simulink model "wind_prili"  (R2021a)
settings: Solver=VariableStepAuto  StartTime=0.0  StopTime=10.0  RelTol=1e-3
undefined symbols (not defined in the file): D1, Delta
libraries: spsThreePhaseVIMeasurementLib x3, spsThreePhaseParallelRLCLoadLib x2, spsPower3phInstantaneousLib x2, spsThreePhaseSourceLib x1, spsExcitationSystemLib x1, spsSynchronousMachinepuStandardLib x1, spsThreePhaseTransformerTwoWindingsLib x1, spsWindTurbineLib x1, spspowerguiLib x1
settings Model: Creator=HP  LastModifiedBy=HP

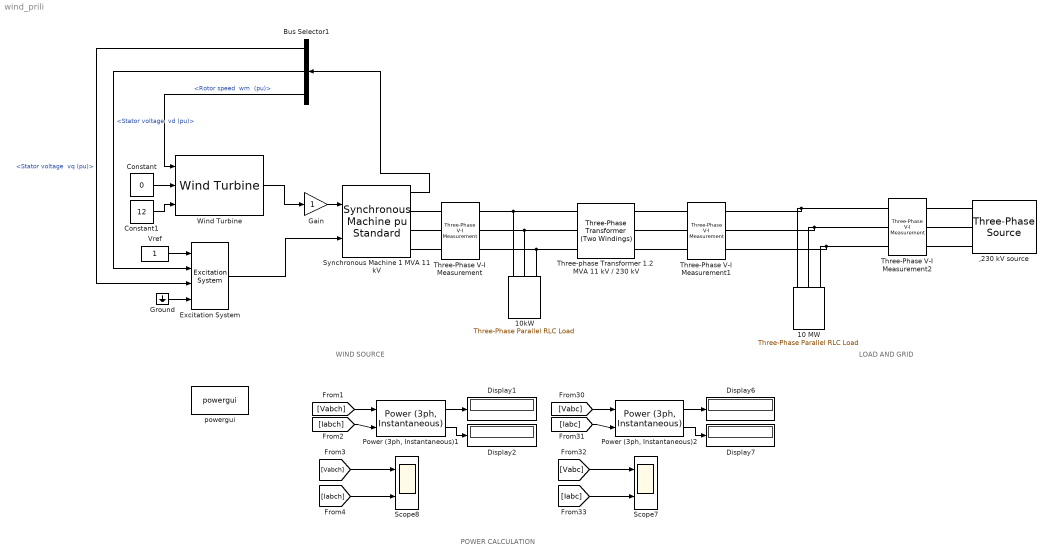
== system wind_prili ==
  note: LOAD AND GRID
  note: WIND SOURCE
  note: POWER CALCULATION
  ,230 kV source : spsThreePhaseSourceLib/Three-Phase Source  InternalConnection=Yg  VoltagePhases=off  Voltage=230e3  PhaseAngle=0  Voltage_phases=[25e3 25e3 25e3]/sqrt(3)  PhaseAngles_phases=[0 -120 +120]  Frequency=50  NonIdealSource=on  SpecifyImpedance=off  Resistance=0.529  Inductance=0.0140  ShortCircuitLevel=10000e6  BaseVoltage=230e3  XRratio=10  BusType=swing  Pref=0  Qref=0  Prefabc=[10e3, 10e3, 10e3]  Qrefabc=[0, 0, 0]  Qmin=-Inf  Qmax=Inf
  10 MW : spsThreePhaseParallelRLCLoadLib/Three-Phase Parallel RLC Load  LConnTagsString=A|B|C  Configuration=Y (grounded)  NominalVoltage=230e3  Vabc=[1e3 1e3 1e3]  Vabcp=[1e3 1e3 1e3]  NominalFrequency=50  UnbalancedPower=off  ActivePower=1.8e6  InductivePower=0.8e6  CapacitivePower=0  Pabc=[10e3 9e3 11e3]  QLabc=[100 90 110]  QCabc=[100 90 110]  Pabcp=[10e3 9e3 11e3]  QLabcp=[100 90 110]  QCabcp=[100 90 110]  Measurements=None  LoadType=constant Z
  10kW : spsThreePhaseParallelRLCLoadLib/Three-Phase Parallel RLC Load  LConnTagsString=A|B|C  Configuration=Y (grounded)  NominalVoltage=11e3  Vabc=[1e3 1e3 1e3]  Vabcp=[1e3 1e3 1e3]  NominalFrequency=50  UnbalancedPower=off  ActivePower=10e3  InductivePower=0  CapacitivePower=0  Pabc=[10e3 9e3 11e3]  QLabc=[100 90 110]  QCabc=[100 90 110]  Pabcp=[10e3 9e3 11e3]  QLabcp=[100 90 110]  QCabcp=[100 90 110]  Measurements=None  LoadType=constant Z
  Bus Selector1 : BusSelector  OutputSignals="dq0 components.Stator voltage  vq (pu),dq0 components.Stator voltage  vd (pu),Mechanical.Rotor speed  wm  (pu)"
  Constant : Constant  Value=0
  Constant1 : Constant  Value=12
  Display{1..2,6..7} (4 alike) : Display
  Excitation System : spsExcitationSystemLib/Excitation System  tr=20e-3  reg=[ 300, 0.001 ]  exc=[ 1, 0 ]  tgr=[ 0, 0 ]  damp=[ 0.001, 0.1 ]  sat=[ 0, 0 ]  lim=[ -11.5, 11.5, 0 ]  v0=[1,1.26864]
      settings: SourceProductBaseCode=PS
  Gain : Gain
  Ground : Ground
  "Power (3ph, Instantaneous)1" : spsPower3phInstantaneousLib/Power (3ph, Instantaneous)
  "Power (3ph, Instantaneous)2" : spsPower3phInstantaneousLib/Power (3ph, Instantaneous)
  Scope7 : Scope  NumInputPorts=2
  Scope8 : Scope  NumInputPorts=2
  Synchronous Machine 1 MVA 11 kV : spsSynchronousMachinepuStandardLib/Synchronous Machine pu Standard  PresetModel=No  MechanicalLoad=Mechanical power Pm  ShowDetailedParameters=on  RotorType=Salient-pole  Units=per unit standard parameters  MeasurementBus=off  NominalParameters="[ 1E6  11e3   50 ]"  Reactances1=[ 31 32 33 34 35 36 37 ]  Reactances2=[ 1.305, 0.296, 0.252, 0.474, 0.243, 0.18 ]  dAxisTimeConstants=Short-circuit  qAxisTimeConstants=Open-circuit  TimeConstants1=[]  TimeConstants2=[]  TimeConstants3=[]  TimeConstants4=[]  TimeConstants5=[ 1.01, 0.053, 0.1 ]  TimeConstants6=[]  TimeConstants7=[]  TimeConstants8=[]  StatorResistance=2.8544e-3  Mechanical=[ 3.2 0 2]  PolePairs=2  InitialConditions=[0 -83.6958 0.750005 0.750005 0.750005 -13.0459 -133.046 106.954 1.26864]  SetSaturation=off  Saturation=[0.6404,0.7127,0.8441,0.9214,0.9956,1.082,1.19,1.316,1.457;0.7,0.7698,0.8872,0.9466,0.9969,1.046,1.1,1.151,1.201]  LoadFlowParameters=[1 150000000 0 0]  TsPowergui=0  TsBlock=-1  IterativeModel=Trapezoidal non iterative  IterativeDiscreteModel=Trapezoidal non iterative  BusType=PV  Pref=150000000  Qref=0  Qmin=-Inf  Qmax=Inf  PLF=0  QLF=0
      settings: SourceProductBaseCode=PS
  Three-Phase V-I Measurement : spsThreePhaseVIMeasurementLib/Three-Phase V-I Measurement  VoltageMeasurement=phase-to-ground  SetLabelV=on  LabelV=Vabc_w  Vpu=off  VpuLL=off  CurrentMeasurement=no  SetLabelI=off  LabelI=Iabc  Ipu=off  Pbase=100e6  Vbase=500e3  OutputType=Complex  PhasorSimulation=off  PSBequivalent=0
  Three-Phase V-I Measurement1 : spsThreePhaseVIMeasurementLib/Three-Phase V-I Measurement  VoltageMeasurement=phase-to-ground  SetLabelV=on  LabelV=Vabch  Vpu=off  VpuLL=off  CurrentMeasurement=yes  SetLabelI=on  LabelI=Iabch  Ipu=off  Pbase=100e6  Vbase=500e3  OutputType=Complex  PhasorSimulation=off  PSBequivalent=0
  Three-Phase V-I Measurement2 : spsThreePhaseVIMeasurementLib/Three-Phase V-I Measurement  VoltageMeasurement=phase-to-ground  SetLabelV=on  LabelV=Vabc  Vpu=off  VpuLL=off  CurrentMeasurement=yes  SetLabelI=on  LabelI=Iabc  Ipu=off  Pbase=100e6  Vbase=500e3  OutputType=Complex  PhasorSimulation=off  PSBequivalent=0
  Three-phase Transformer 1.2 MVA 11 kV / 230 kV : spsThreePhaseTransformerTwoWindingsLib/Three-Phase Transformer (Two Windings)  Winding1Connection=Delta (D1)  Winding2Connection=Yg  CoreType=Three single-phase transformers  SetSaturation=off  Hysteresis=off  DataFile='hysteresis'  SetInitialFlux=off  Measurements=None  UNITS=pu  NominalPower=[ 1.2e6 50 ]  Winding1="[ 11e3 0.0027  0.08]"  Winding2=[ 230e3 0.0027 0.08]  Rm=500  Lm=500  L0=0.5  Saturation="[ 0,0  ;  0.005,1.2  ;  1.0,1.4 ]"  InitialFluxes=[ 0.8 , -0.8 , 0.7 ]  BreakLoop=off  DiscreteSolver=Trapezoidal iterative  DataType=off  TransfoNumber=0
  Vref : Constant
  Wind Turbine : spsWindTurbineLib/Wind Turbine  Pnom=10e6  Pelec_base=10e6/0.9  wind_base=12  P_wind_base=0.8  speed_nom=1.2  pitch_angle=0  c1_c6="[0.51763          116          0.4            5           21     0.006795]"  cp_nom=0.48  lambda_nom=8.1
      link override Gain: Gain=1
      settings: SourceProductBaseCode=PS
  powergui : spspowerguiLib/powergui  Priority=2  SimulationMode=Continuous  SampleTime=0  frequency=60  Iterations=50  frequencyindice=50  Pbase=100e6  ErrMax=0.0001  UnitsV=kV  UnitsW=MW  buscounter=0  FunctionMessages=off  echomessages=off  EnableUseOfTLC=off  CurrentSourceSwitches=off  DisableSnubberDevices=off  DisableRonSwitches=off  DisableVfSwitches=off  DisplayEquations=off  AutomaticDiscreteSolvers=off  SolverType=Tustin  Interpol=off  ExternalGateDelay=off  methode=off  Ts=0  x0status=blocks  SPID=on  SwTol=0  HookPort=off  NonlinearTolerance=1e-4  nMaxIteration=100  ContinueOnMaxIteration=off  RestoreLinks=warning  ResistiveCurrentMeasurement=off  Frange=logspace(0,3,50)  Ylog=off  Xlog=off  ShowGrid=off  save=off  variable=ZData  structure=0  ZoomFFT=on  StartTime=0.0  cycles=2  DisplayStyle=off  fundamental=60  FreqAxis=off  MaxFrequency=1000  frequencyindicesteady=1  RmsSteady=1  display=off
  wires:
  [Vabc] -> Scope7/1
  "Power (3ph, Instantaneous)2"/1 -> Display6/1
  "Power (3ph, Instantaneous)1"/2 -> Display2/1
  [Vabc] -> "Power (3ph, Instantaneous)2"/1
  [Iabc] -> Scope7/2
  Bus Selector1/1 -> Excitation System/3  "<Stator voltage  vq (pu)>"
  "Power (3ph, Instantaneous)2"/2 -> Display7/1
  Ground/1 -> Excitation System/4
  [Vabch] -> Scope8/1
  Excitation System/1 -> Synchronous Machine 1 MVA 11 kV/2
  [Iabch] -> Scope8/2
  [Iabch] -> "Power (3ph, Instantaneous)1"/2
  Synchronous Machine 1 MVA 11 kV/1 -> Bus Selector1/1
  "Power (3ph, Instantaneous)1"/1 -> Display1/1
  [Iabc] -> "Power (3ph, Instantaneous)2"/2
  Bus Selector1/2 -> Excitation System/2  "<Stator voltage  vd (pu)>"
  [Vabch] -> "Power (3ph, Instantaneous)1"/1
  Vref/1 -> Excitation System/1
  Bus Selector1/3 -> Wind Turbine/1  "<Rotor speed  wm  (pu)>"
  Constant/1 -> Wind Turbine/2
  Constant1/1 -> Wind Turbine/3
  Gain/1 -> Synchronous Machine 1 MVA 11 kV/1
  Wind Turbine/1 -> Gain/1
  connections:
  Three-Phase V-I Measurement/RConn1 -- 10kW/LConn1 -- Three-phase Transformer 1.2 MVA 11 kV / 230 kV/LConn1
  Three-Phase V-I Measurement/RConn3 -- 10kW/LConn3 -- Three-phase Transformer 1.2 MVA 11 kV / 230 kV/LConn3
  10 MW/LConn3 -- Three-Phase V-I Measurement1/RConn3 -- Three-Phase V-I Measurement2/RConn3
  Three-Phase V-I Measurement/RConn2 -- 10kW/LConn2 -- Three-phase Transformer 1.2 MVA 11 kV / 230 kV/LConn2
  10 MW/LConn1 -- Three-Phase V-I Measurement1/RConn1 -- Three-Phase V-I Measurement2/RConn1
  10 MW/LConn2 -- Three-Phase V-I Measurement1/RConn2 -- Three-Phase V-I Measurement2/RConn2
  Synchronous Machine 1 MVA 11 kV/RConn2 -- Three-Phase V-I Measurement/LConn2
  Three-Phase V-I Measurement2/LConn1 -- ,230 kV source/RConn1
  Three-Phase V-I Measurement2/LConn3 -- ,230 kV source/RConn3
  Three-Phase V-I Measurement1/LConn3 -- Three-phase Transformer 1.2 MVA 11 kV / 230 kV/RConn3
  Three-Phase V-I Measurement2/LConn2 -- ,230 kV source/RConn2
  Three-Phase V-I Measurement1/LConn1 -- Three-phase Transformer 1.2 MVA 11 kV / 230 kV/RConn1
  Three-Phase V-I Measurement1/LConn2 -- Three-phase Transformer 1.2 MVA 11 kV / 230 kV/RConn2
  Synchronous Machine 1 MVA 11 kV/RConn1 -- Three-Phase V-I Measurement/LConn1
  Synchronous Machine 1 MVA 11 kV/RConn3 -- Three-Phase V-I Measurement/LConn3
